simulink model "DR_ForceToTorque"  (R2022a)
settings: Solver=VariableStepAuto  StartTime=0.0  StopTime=10  RelTol=1e-3
undefined symbols (not defined in the file): X, Y, Z
libraries: sm_lib x9, nesl_utility x7
settings Model: Creator=bobjo  LastModifiedBy=bobjo

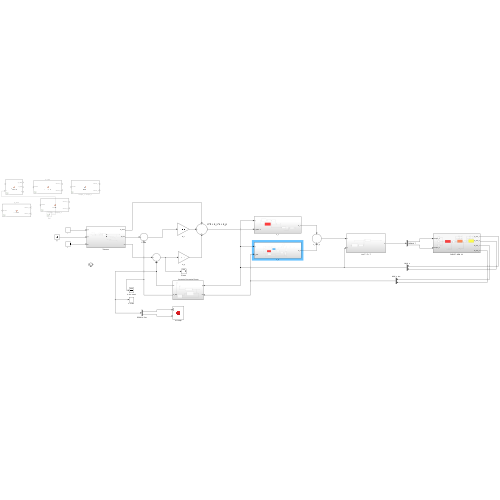
[thumbnail: Simulink's stored preview of the top-level diagram]
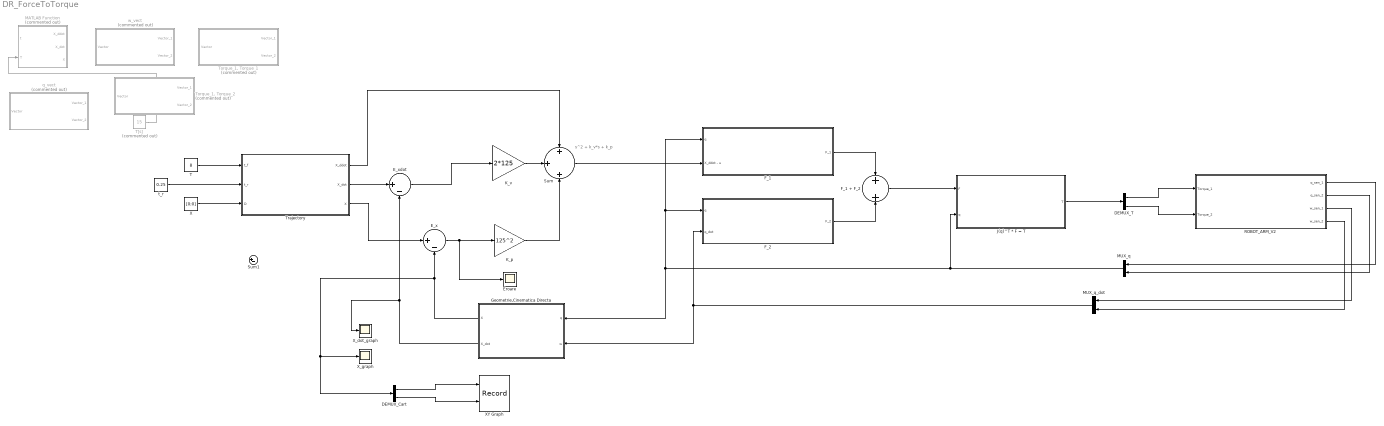
== system DR_ForceToTorque ==
  note: s^2 + k_v*s + k_p
  " MUX_q" : Mux  Inputs=2
  DEMUX_Cart : Demux  Outputs=2
  DEMUX_T : Demux  Outputs=2
  E_x : Sum  Inputs=|+-
  E_xdot : Sum  Inputs=|+-
  Eroare : Scope
  F_1 : Subsystem
  F_1 + F_2 : Sum  Inputs=+|+
  F_2 : Subsystem
  Geometrie,Cinematica Directa : Subsystem
  J(q)^T * F = T : Subsystem
  K_p : Gain  Gain=125^2
  K_v : Gain  Gain=2*125
  MATLAB Function : MATLAB Function  Commented=on  TreatAsAtomicUnit=on
  MUX_q_dot : Mux  Inputs=2
  ROBOT_ARM_V2 : Subsystem
  Sum : Sum  Inputs=+|+|+
  Sum1 : Sum  Inputs=|+-
  T : Constant  Value=8
  T[s] : Constant  Commented=on  Value=15
  "Torque_1, Torque_1" : MATLAB Function  Commented=on  TreatAsAtomicUnit=on
  "Torque_1, Torque_2" : MATLAB Function  Commented=on  TreatAsAtomicUnit=on
  Trajectory : Subsystem
  X : Constant  Value=[0;0]
  XY Graph : Record  FileSettingsInternal="{\"entries\":[{\"content\":{\"excelSettings\":{\"content\":{},\"type\":\"Streamout.ExcelSettings\"}},\"type\":\"Streamout.FileSettingStorage\",\"uuid\":\"b94b4cba-0fe7-4e66-af93-bfd95075920f\"}],\"packageUris\":[\"http://schema.mathworks.com/mf0/streamout_blocks/R2020a\"],\"version\":\"1.0\"}"  Layout=[1 1]  SignalsInternal="{\"entries\":[{\"content\":{\"signals\":[{\"content\":{\"blockPath\":[\"DR_ForceToTorque/XY Graph\"],\"channel\":[],\"dimensions\":[1,1],\"domain\":\"DR_ForceToTorque/XY Graph\",\"lineColor\":\"#a2142f\",\"plots\":[1],\"port\":1,\"sid\":[\"\"],\"signalID\":20,\"signalName\":\"DEMUX_Cart:1\"},\"type\":\"RecordBlkView.Signal\",\"uuid\":\"102e7f18-ab4c-4a7b-a2e7-68a635edeffb\"},{\"content\":{\"blockPath\":[\"DR_ForceToTorque/XY Graph\"],\"channel\":[],\"dimensions\":[1,1],\"domain\":\"DR_ForceToTorque/XY Graph\",\"lineColor\":\"#139fff\",\"plots\":[1],\"port\":2,\"sid\":[\"\"],\"signalID\":24,\"signalName\":\"DEMUX_Cart:2\"},\"type\":\"RecordBlkView.Signal\",\"uuid\":\"6c0b5dfe-2c0c-4a8d-93c7-f0d4dc18e998\"}]},\"type\":\"RecordBlkView.InputSignals\",\"uuid\":\"2a78a68b-d20b-47b5-ae5b-fe216d435864\"}],\"packageUris\":[\"http://schema.mathworks.com/mf0/streamout_blocks/R2020a\"],\"version\":\"1.0\"}"  VisualizationBindings="{\"xyplotplugin\":{\"info\":[{\"series\":[{\"bindingParametersList\":[{\"parameter\":\"X-Axis\",\"signalID\":20,\"signalName\":\"DEMUX_Cart:1\"},{\"parameter\":\"Y-Axis\",\"signalID\":24,\"signalName\":\"DEMUX_Cart:2\"}],\"seriesID\":43765}],\"subplotID\":1}]}}"  CompatibilityTag=XY
  X_dot_graph : Scope
  X_graph : Scope
  q_vect : MATLAB Function  Commented=on  TreatAsAtomicUnit=on
  t_r : Constant  Value=0.25
  w_vect : MATLAB Function  Commented=on  TreatAsAtomicUnit=on
  wires:
  F_1/1(F_1) -> F_1 + F_2/1
  F_2/1(F_2) -> F_1 + F_2/2
  F_1 + F_2/1 -> J(q)^T * F = T/1(F)
  Sum/1 -> F_1/2(X_ddot - u)
  E_x/1 -> Eroare/1, K_p/1
  E_xdot/1 -> K_v/1
  K_v/1 -> Sum/2
  K_p/1 -> Sum/3
  Geometrie,Cinematica Directa/2(X_dot) -> X_dot_graph/1, E_xdot/2
  Geometrie,Cinematica Directa/1(X) -> DEMUX_Cart/1, X_graph/1, E_x/2
  T[s]/1 -> MATLAB Function/2(T)
  T/1 -> Trajectory/1("t_f ")
  t_r/1 -> Trajectory/2("t_r ")
  Trajectory/1(X_ddot) -> Sum/1
  Trajectory/2(X_dot) -> E_xdot/1
  Trajectory/3(X) -> E_x/1
  J(q)^T * F = T/1(T) -> DEMUX_T/1
  DEMUX_T/1 -> ROBOT_ARM_V2/1(Torque_1)
  DEMUX_T/2 -> ROBOT_ARM_V2/2(Torque_2)
  ROBOT_ARM_V2/1(q_sen_1) -> " MUX_q"/1
  ROBOT_ARM_V2/2(q_sen_2) -> " MUX_q"/2
  ROBOT_ARM_V2/3(w_sen_1) -> MUX_q_dot/1
  ROBOT_ARM_V2/4(w_sen_2) -> MUX_q_dot/2
  " MUX_q"/1 -> Geometrie,Cinematica Directa/1(q), F_1/1(q), F_2/1(q), J(q)^T * F = T/2(q)
  MUX_q_dot/1 -> Geometrie,Cinematica Directa/2(w), F_2/2(q_dot)
  DEMUX_Cart/1 -> XY Graph/1
  DEMUX_Cart/2 -> XY Graph/2
  X/1 -> Trajectory/3(D)

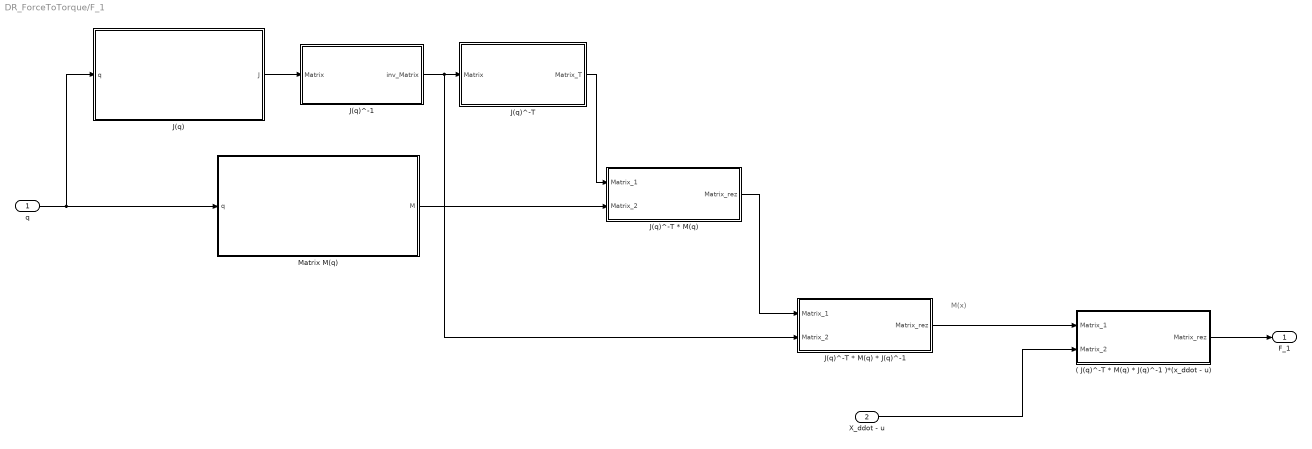
== system DR_ForceToTorque/F_1 ==
  note: M(x)
  q : Inport
  X_ddot - u : Inport  Port=2
  ( J(q)^-T * M(q) * J(q)^-1 )*(x_ddot - u) : MATLAB Function  TreatAsAtomicUnit=on
  J(q) : MATLAB Function  TreatAsAtomicUnit=on
  J(q)^-1 : MATLAB Function  TreatAsAtomicUnit=on
  J(q)^-T : MATLAB Function  TreatAsAtomicUnit=on
  J(q)^-T * M(q) : MATLAB Function  TreatAsAtomicUnit=on
  J(q)^-T * M(q) * J(q)^-1 : MATLAB Function  TreatAsAtomicUnit=on
  Matrix M(q) : MATLAB Function  TreatAsAtomicUnit=on
  F_1 : Outport
  wires:
  Matrix M(q)/1(M) -> J(q)^-T * M(q)/2(Matrix_2)
  J(q)/1(J) -> J(q)^-1/1(Matrix)
  J(q)^-1/1(inv_Matrix) -> J(q)^-T/1(Matrix), J(q)^-T * M(q) * J(q)^-1/2(Matrix_2)
  ( J(q)^-T * M(q) * J(q)^-1 )*(x_ddot - u)/1(Matrix_rez) -> F_1/1
  q/1 -> Matrix M(q)/1(q), J(q)/1(q)
  J(q)^-T * M(q)/1(Matrix_rez) -> J(q)^-T * M(q) * J(q)^-1/1(Matrix_1)
  J(q)^-T * M(q) * J(q)^-1/1(Matrix_rez) -> ( J(q)^-T * M(q) * J(q)^-1 )*(x_ddot - u)/1(Matrix_1)
  X_ddot - u/1 -> ( J(q)^-T * M(q) * J(q)^-1 )*(x_ddot - u)/2(Matrix_2)
  J(q)^-T/1(Matrix_T) -> J(q)^-T * M(q)/1(Matrix_1)

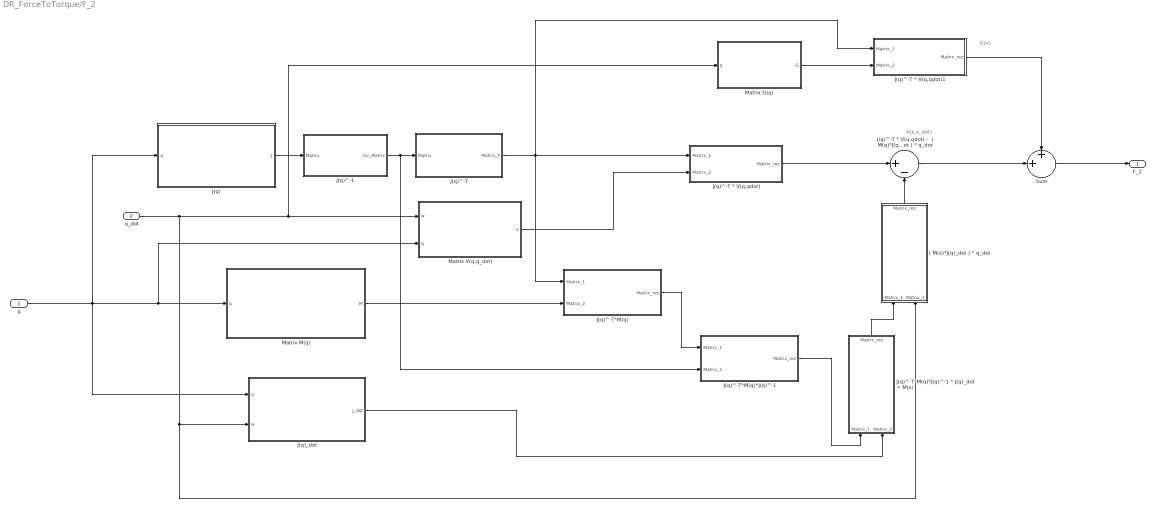
== system DR_ForceToTorque/F_2 ==
  note: G(x)
  note: V(x,x_dot)
  q : Inport
  q_dot : Inport  Port=2
  ( M(x)*J(q)_dot ) * q_dot : MATLAB Function  TreatAsAtomicUnit=on
  J(q) : MATLAB Function  TreatAsAtomicUnit=on
  J(q)^-1 : MATLAB Function  TreatAsAtomicUnit=on
  J(q)^-T : MATLAB Function  TreatAsAtomicUnit=on
  J(q)^-T * V(q,qdot) : MATLAB Function  TreatAsAtomicUnit=on
  J(q)^-T * V(q,qdot) -  ( M(q)*J(q)_dot ) * q_dot : Sum  Inputs=|+-
  J(q)^-T * V(q,qdot)1 : MATLAB Function  TreatAsAtomicUnit=on
  J(q)^-T*M(q) : MATLAB Function  TreatAsAtomicUnit=on
  J(q)^-T*M(q)*J(q)^-1 : MATLAB Function  TreatAsAtomicUnit=on
  J(q)^-T*M(q)*J(q)^-1 * J(q)_dot = M(x) : MATLAB Function  TreatAsAtomicUnit=on
  J(q)_dot : MATLAB Function  TreatAsAtomicUnit=on
  Matrix G(q) : MATLAB Function  TreatAsAtomicUnit=on
  Matrix M(q) : MATLAB Function  TreatAsAtomicUnit=on
  Matrix V(q,q_dot) : MATLAB Function  TreatAsAtomicUnit=on
  Sum : Sum  Inputs=++|
  F_2 : Outport
  wires:
  q/1 -> J(q)/1(q), J(q)_dot/1(q), Matrix V(q,q_dot)/2(q), Matrix M(q)/1(q)
  J(q)/1(J) -> J(q)^-1/1(Matrix)
  J(q)^-1/1(inv_Matrix) -> J(q)^-T/1(Matrix), J(q)^-T*M(q)*J(q)^-1/2(Matrix_2)
  J(q)^-T/1(Matrix_T) -> J(q)^-T * V(q,qdot)/1(Matrix_1), J(q)^-T * V(q,qdot)1/1(Matrix_1), J(q)^-T*M(q)/1(Matrix_1)
  Matrix V(q,q_dot)/1(V) -> J(q)^-T * V(q,qdot)/2(Matrix_2)
  q_dot/1 -> J(q)_dot/2(w), ( M(x)*J(q)_dot ) * q_dot/2(Matrix_2), Matrix G(q)/1(q), Matrix V(q,q_dot)/1(w)
  J(q)^-T * V(q,qdot)/1(Matrix_rez) -> J(q)^-T * V(q,qdot) -  ( M(q)*J(q)_dot ) * q_dot/1
  J(q)_dot/1(J_dot) -> J(q)^-T*M(q)*J(q)^-1 * J(q)_dot = M(x)/2(Matrix_2)
  J(q)^-T*M(q)*J(q)^-1 * J(q)_dot = M(x)/1(Matrix_rez) -> ( M(x)*J(q)_dot ) * q_dot/1(Matrix_1)
  ( M(x)*J(q)_dot ) * q_dot/1(Matrix_rez) -> J(q)^-T * V(q,qdot) -  ( M(q)*J(q)_dot ) * q_dot/2
  Matrix M(q)/1(M) -> J(q)^-T*M(q)/2(Matrix_2)
  J(q)^-T*M(q)/1(Matrix_rez) -> J(q)^-T*M(q)*J(q)^-1/1(Matrix_1)
  J(q)^-T*M(q)*J(q)^-1/1(Matrix_rez) -> J(q)^-T*M(q)*J(q)^-1 * J(q)_dot = M(x)/1(Matrix_1)
  Sum/1 -> F_2/1
  J(q)^-T * V(q,qdot) -  ( M(q)*J(q)_dot ) * q_dot/1 -> Sum/2
  Matrix G(q)/1(G) -> J(q)^-T * V(q,qdot)1/2(Matrix_2)
  J(q)^-T * V(q,qdot)1/1(Matrix_rez) -> Sum/1

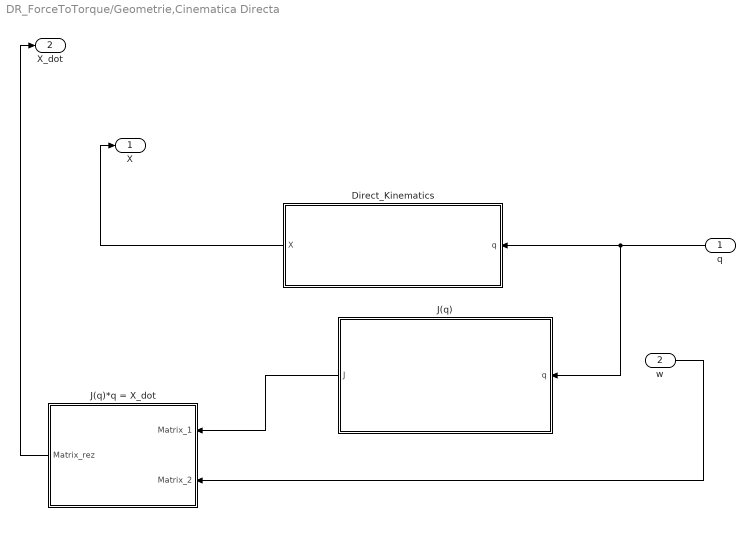
== system DR_ForceToTorque/Geometrie,Cinematica Directa ==
  q : Inport
  w : Inport  Port=2
  Direct_Kinematics : MATLAB Function  TreatAsAtomicUnit=on
  J(q) : MATLAB Function  TreatAsAtomicUnit=on
  J(q)*q = X_dot : MATLAB Function  TreatAsAtomicUnit=on
  X : Outport
  X_dot : Outport  Port=2
  wires:
  w/1 -> J(q)*q = X_dot/2(Matrix_2)
  Direct_Kinematics/1(X) -> X/1
  J(q)/1(J) -> J(q)*q = X_dot/1(Matrix_1)
  q/1 -> J(q)/1(q), Direct_Kinematics/1(q)
  J(q)*q = X_dot/1(Matrix_rez) -> X_dot/1

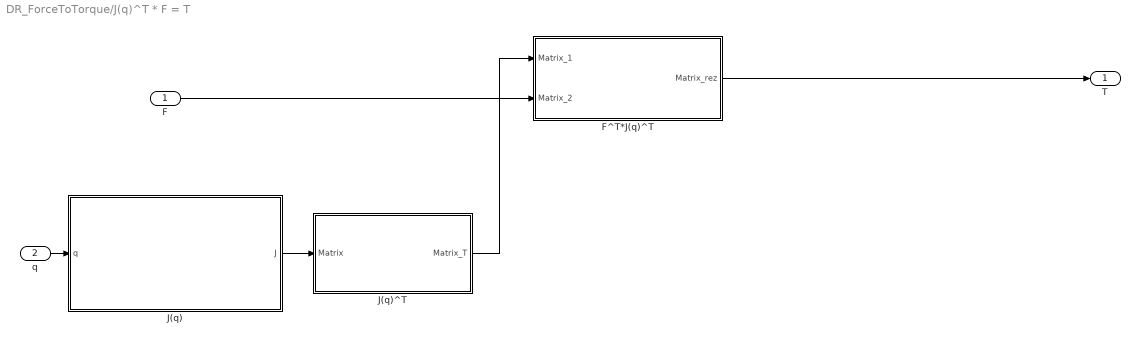
== system DR_ForceToTorque/J(q)^T * F = T ==
  F : Inport
  q : Inport  Port=2
  F^T*J(q)^T : MATLAB Function  TreatAsAtomicUnit=on
  J(q) : MATLAB Function  TreatAsAtomicUnit=on
  J(q)^T : MATLAB Function  TreatAsAtomicUnit=on
  T : Outport
  wires:
  J(q)/1(J) -> J(q)^T/1(Matrix)
  q/1 -> J(q)/1(q)
  J(q)^T/1(Matrix_T) -> F^T*J(q)^T/1(Matrix_1)
  F^T*J(q)^T/1(Matrix_rez) -> T/1
  F/1 -> F^T*J(q)^T/2(Matrix_2)

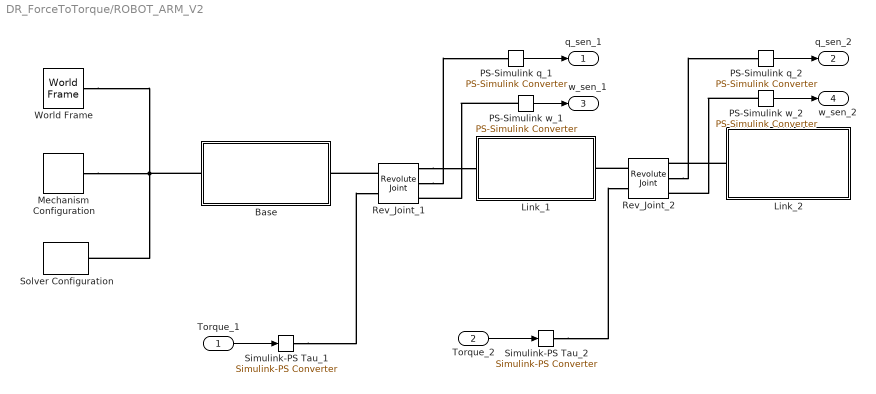
== system DR_ForceToTorque/ROBOT_ARM_V2 ==
  Torque_1 : Inport
  Torque_2 : Inport  Port=2
  Base : Subsystem
  Link_1 : Subsystem
  Link_2 : Subsystem
  Mechanism Configuration : sm_lib/Utilities/Mechanism Configuration  UniformGravity=Constant  GravityVector=[0 0 -9.80665]  GravityUnits=m/s^2  LinearizationDelta=0.001  JointModeTransitionNonlinearIterations=2
  PS-Simulink q_1 : nesl_utility/PS-Simulink Converter  PhysicalDomain=network_engine_domain  SubClassName=ps_output  LeftPortType=input  RightPortType=output  PseudoPeriodic=off  Frequencies=[]  VectorFormat=inherit  Unit=inherit  AffineConversion=off
      settings: SourceProductBaseCode=SS,PW,VE
  PS-Simulink q_2 : nesl_utility/PS-Simulink Converter  PhysicalDomain=network_engine_domain  SubClassName=ps_output  LeftPortType=input  RightPortType=output  PseudoPeriodic=off  Frequencies=[]  VectorFormat=inherit  Unit=inherit  AffineConversion=off
      settings: SourceProductBaseCode=SS,PW,VE
  PS-Simulink w_1 : nesl_utility/PS-Simulink Converter  PhysicalDomain=network_engine_domain  SubClassName=ps_output  LeftPortType=input  RightPortType=output  PseudoPeriodic=off  Frequencies=[]  VectorFormat=inherit  Unit=inherit  AffineConversion=off
      settings: SourceProductBaseCode=SS,PW,VE
  PS-Simulink w_2 : nesl_utility/PS-Simulink Converter  PhysicalDomain=network_engine_domain  SubClassName=ps_output  LeftPortType=input  RightPortType=output  PseudoPeriodic=off  Frequencies=[]  VectorFormat=inherit  Unit=inherit  AffineConversion=off
      settings: SourceProductBaseCode=SS,PW,VE
  Rev_Joint_1 : sm_lib/Joints/Revolute Joint  JointMode=Normal  SenseConstraintForce=off  SenseConstraintForceX=off  SenseConstraintForceY=off  SenseConstraintForceZ=off  SenseConstraintTorque=off  SenseConstraintTorqueX=off  SenseConstraintTorqueY=off  SenseConstraintTorqueZ=off  SenseTotalForce=off  SenseTotalForceX=off  SenseTotalForceY=off  SenseTotalForceZ=off  SenseTotalTorque=off  SenseTotalTorqueX=off  SenseTotalTorqueY=off  SenseTotalTorqueZ=off  CompositeWrenchDir=FollowerOnBase  CompositeWrenchFrame=BaseFrame  EquilibriumPosition=0  EquilibriumPositionUnits=deg  SpringStiffness=0  SpringStiffnessUnits=N*m/deg  DampingCoefficient=0  DampingCoefficientUnits=N*m/(deg/s)  TorqueActuationMode=InputTorque  MotionActuationMode=ComputedMotion  SensePosition=on  SenseVelocity=on  SenseAcceleration=off  SenseTorqueForce=off  SenseLowerLimitTorqueForce=off  SenseUpperLimitTorqueForce=off  LowerLimitSpecify=off  LowerLimitBound=-90  LowerLimitBoundUnits=deg  LowerLimitStiffness=1e4  LowerLimitStiffnessUnits=N*m/deg  LowerLimitDamping=10  LowerLimitDampingUnits=N*m/(deg/s)  LowerLimitTransitionRegionWidth=0.1  LowerLimitTransitionRegionWidthUnits=deg  UpperLimitSpecify=off  UpperLimitBound=90  UpperLimitBoundUnits=deg  UpperLimitStiffness=1e4  UpperLimitStiffnessUnits=N*m/deg  UpperLimitDamping=10  UpperLimitDampingUnits=N*m/(deg/s)  UpperLimitTransitionRegionWidth=0.1  UpperLimitTransitionRegionWidthUnits=deg  PositionTargetSpecify=on  PositionTargetPriority=High  PositionTargetValue=0  PositionTargetValueUnits=rad  VelocityTargetSpecify=off  VelocityTargetPriority=High  VelocityTargetValue=0  VelocityTargetValueUnits=deg/s
  Rev_Joint_2 : sm_lib/Joints/Revolute Joint  JointMode=Normal  SenseConstraintForce=off  SenseConstraintForceX=off  SenseConstraintForceY=off  SenseConstraintForceZ=off  SenseConstraintTorque=off  SenseConstraintTorqueX=off  SenseConstraintTorqueY=off  SenseConstraintTorqueZ=off  SenseTotalForce=off  SenseTotalForceX=off  SenseTotalForceY=off  SenseTotalForceZ=off  SenseTotalTorque=off  SenseTotalTorqueX=off  SenseTotalTorqueY=off  SenseTotalTorqueZ=off  CompositeWrenchDir=FollowerOnBase  CompositeWrenchFrame=BaseFrame  EquilibriumPosition=0  EquilibriumPositionUnits=deg  SpringStiffness=0  SpringStiffnessUnits=N*m/deg  DampingCoefficient=0  DampingCoefficientUnits=N*m/(deg/s)  TorqueActuationMode=InputTorque  MotionActuationMode=ComputedMotion  SensePosition=on  SenseVelocity=on  SenseAcceleration=off  SenseTorqueForce=off  SenseLowerLimitTorqueForce=off  SenseUpperLimitTorqueForce=off  LowerLimitSpecify=off  LowerLimitBound=-90  LowerLimitBoundUnits=deg  LowerLimitStiffness=1e4  LowerLimitStiffnessUnits=N*m/deg  LowerLimitDamping=10  LowerLimitDampingUnits=N*m/(deg/s)  LowerLimitTransitionRegionWidth=0.1  LowerLimitTransitionRegionWidthUnits=deg  UpperLimitSpecify=off  UpperLimitBound=90  UpperLimitBoundUnits=deg  UpperLimitStiffness=1e4  UpperLimitStiffnessUnits=N*m/deg  UpperLimitDamping=10  UpperLimitDampingUnits=N*m/(deg/s)  UpperLimitTransitionRegionWidth=0.1  UpperLimitTransitionRegionWidthUnits=deg  PositionTargetSpecify=on  PositionTargetPriority=High  PositionTargetValue=0  PositionTargetValueUnits=rad  VelocityTargetSpecify=off  VelocityTargetPriority=High  VelocityTargetValue=0  VelocityTargetValueUnits=deg/s
  Simulink-PS Tau_1 : nesl_utility/Simulink-PS Converter  PhysicalDomain=network_engine_domain  SubClassName=ps_input  LeftPortType=input  RightPortType=output  PseudoPeriodic=off  Frequencies=[]  NoiseDistribution=none  NoiseParameters=[]  Unit=N*m  AffineConversion=off  FilteringAndDerivatives=provide  SimscapeFilterOrder=2  InputFilterTimeConstant=0.001  UdotUserProvided=0
      settings: SourceProductBaseCode=SS,PW,VE
  Simulink-PS Tau_2 : nesl_utility/Simulink-PS Converter  PhysicalDomain=network_engine_domain  SubClassName=ps_input  LeftPortType=input  RightPortType=output  PseudoPeriodic=off  Frequencies=[]  NoiseDistribution=none  NoiseParameters=[]  Unit=N*m  AffineConversion=off  FilteringAndDerivatives=provide  SimscapeFilterOrder=2  InputFilterTimeConstant=0.001  UdotUserProvided=0
      settings: SourceProductBaseCode=SS,PW,VE
  Solver Configuration : nesl_utility/Solver Configuration  PhysicalDomain=network_engine_domain  SubClassName=solver  LeftPortType=input  RightPortType=generic  Tones=[]  Harmonics=[]  SimulateNoise=off  Profile=off  UseLocalSampling=off  EnableSwitchedLinearOptims=on  FrequencyDomain=off  UseCCode=off  RelTol=0.001  AbsTol=0.001  MinStep=1e-09  ToWorkspace=off  RevertToSquareIcSolve=off  NumHomotopyIterations=100  PhasorMode=off  PhasorModeNumHarmonics=1  IndexReductionMethod=DerivativeReplacement  DoDC=off  ResidualTolerance=1e-09  UseLocalSolver=off  LocalSolverChoice=NE_BACKWARD_EULER_ADVANCER  LocalSolverSampleTime=0.001  DoFixedCost=off  MaxNonlinIter=3  MaxModeIter=2  ComputeImpulses=off  ImpulseIterations=2  LinearAlgebra=auto  LinearAlgebraNumThread=0  EquationFormulation=NE_TIME_EF  DelaysMemoryBudget=1024  AutomaticFiltering=on  FilteringTimeConstant=0.001  PartitionStorageMethod=AS_NEEDED  PartitionMemoryBudget=1024  PartitionMethod=ROBUST
      settings: SourceProductBaseCode=SS,PW,VE
  World Frame : sm_lib/Frames and Transforms/World Frame
  q_sen_1 : Outport
  q_sen_2 : Outport  Port=2
  w_sen_1 : Outport  Port=3
  w_sen_2 : Outport  Port=4
  wires:
  Torque_1/1 -> Simulink-PS Tau_1/1
  Torque_2/1 -> Simulink-PS Tau_2/1
  PS-Simulink q_1/1 -> q_sen_1/1
  PS-Simulink q_2/1 -> q_sen_2/1
  PS-Simulink w_1/1 -> w_sen_1/1
  PS-Simulink w_2/1 -> w_sen_2/1
  connections:
  Rev_Joint_2/RConn2 -- PS-Simulink q_2/LConn1
  Simulink-PS Tau_1/RConn1 -- Rev_Joint_1/LConn2
  Simulink-PS Tau_2/RConn1 -- Rev_Joint_2/LConn2
  Mechanism Configuration/RConn1 -- Solver Configuration/RConn1 -- Base/LConn1 -- World Frame/RConn1
  Rev_Joint_1/LConn1 -- Base/RConn1
  Rev_Joint_1/RConn1 -- Link_1/LConn1
  Rev_Joint_2/LConn1 -- Link_1/RConn1
  Rev_Joint_1/RConn2 -- PS-Simulink q_1/LConn1
  Link_2/RConn1 -- Rev_Joint_2/RConn1
  PS-Simulink w_2/LConn1 -- Rev_Joint_2/RConn3
  PS-Simulink w_1/LConn1 -- Rev_Joint_1/RConn3

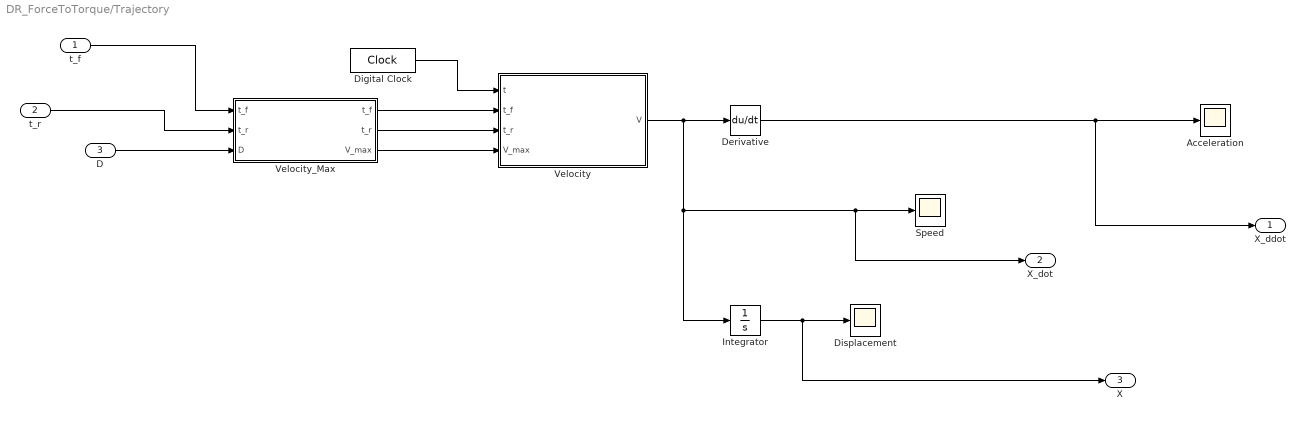
== system DR_ForceToTorque/Trajectory ==
  "t_f " : Inport
  "t_r " : Inport  Port=2
  D : Inport  Port=3
  Acceleration : Scope
  Derivative : Derivative
  Digital Clock : DigitalClock  SampleTime=0.001
  Displacement : Scope
  Integrator : Integrator  InitialCondition=[1;0]
  Speed : Scope
  Velocity : MATLAB Function  TreatAsAtomicUnit=on
  Velocity_Max : MATLAB Function  TreatAsAtomicUnit=on
  X_ddot : Outport
  X_dot : Outport  Port=2
  X : Outport  Port=3
  wires:
  Velocity/1(V) -> X_dot/1, Speed/1, Integrator/1, Derivative/1
  Digital Clock/1 -> Velocity/1(t)
  Integrator/1 -> Displacement/1, X/1
  Derivative/1 -> Acceleration/1, X_ddot/1
  "t_f "/1 -> Velocity_Max/1("t_f ")
  Velocity_Max/1(t_f) -> Velocity/2(t_f)
  Velocity_Max/3(V_max) -> Velocity/4(V_max)
  "t_r "/1 -> Velocity_Max/2("t_r ")
  Velocity_Max/2(t_r) -> Velocity/3(t_r)
  D/1 -> Velocity_Max/3(D)

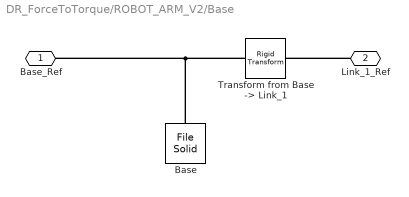
== system DR_ForceToTorque/ROBOT_ARM_V2/Base ==
  Base : sm_lib/Body Elements/File Solid  ExtGeomFileName=C:\Users\bobjo\OneDrive\Desktop\Facultate ROBO\Anul III\DR\Base_V2.CATPart  UnitType=FromFile  ExtGeomFileUnits=m  StepReaderType=HEX  ExportConvexHullGeometry=off  InertiaType=CalculateFromGeometry  Mass=1  MassUnits=kg  CenterOfMass=[0 0 0]  CenterOfMassUnits=m  MomentsOfInertia=[1 1 1]  MomentsOfInertiaUnits=kg*m^2  ProductsOfInertia=[0 0 0]  ProductsOfInertiaUnits=kg*m^2  BasedOnType=DensityFromFile  Density=1000  DensityUnits=kg/m^3  DoExposeReferenceFrame=on  SerializedFrames=<Frames/>  GraphicType=FromGeometry  MarkerShape=Sphere  MarkerSize=10  GraphicVisPropType=SimpleVisualProperties  GraphicDiffuseColor=[1.0 0.0 0.2]  GraphicSpecularColor=[0.5 0.5 0.5 1.0]  GraphicAmbientColor=[0.15 0.15 0.15 1.0]  GraphicEmissiveColor=[0.0 0.0 0.0 1.0]  GraphicShininess=75  GraphicOpacity=1.0
  "Transform from Base -> Link_1" : sm_lib/Frames and Transforms/Rigid Transform  TranslationMethod=Cartesian  TranslationStandardOffset=0  TranslationLengthUnit=mm  TranslationStandardAxis=+Z  TranslationCartesianOffset=[0 0 40]  TranslationROffset=0  TranslationROffsetUnits=m  TranslationZOffset=0  TranslationZOffsetUnits=m  TranslationThetaOffset=0  TranslationThetaOffsetUnits=deg  RotationMethod=None  RotationAngleUnits=deg  RotationStandardAxis=+Z  RotationAngle=0.0  RotationArbitraryAxis=[0 0 1]  FollAlignAxisA=+X  BaseAlignAxisA=+Y  FollAlignAxisB=+Y  BaseAlignAxisB=+Z  RotationSequenceAxes=FollowerAxes  RotationSequence=XYX  RotationSequenceAngles=[0 0 0]  RotationSequenceAnglesUnits=deg  RotationMatrix=[1 0 0; 0 1 0; 0 0 1]
  Base_Ref : PMIOPort  Side=Left
  Link_1_Ref : PMIOPort  Port=2  Side=Right
  connections:
  Base/RConn1 -- Base_Ref/RConn1 -- "Transform from Base -> Link_1"/LConn1
  Link_1_Ref/RConn1 -- "Transform from Base -> Link_1"/RConn1

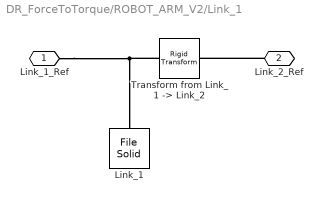
== system DR_ForceToTorque/ROBOT_ARM_V2/Link_1 ==
  Link_1 : sm_lib/Body Elements/File Solid  ExtGeomFileName=C:\Users\bobjo\OneDrive\Desktop\Facultate ROBO\Anul III\DR\Link_1_V2.CATPart  UnitType=FromFile  ExtGeomFileUnits=m  StepReaderType=HEX  ExportConvexHullGeometry=off  InertiaType=CalculateFromGeometry  Mass=0.25  MassUnits=kg  CenterOfMass=[0 0 0]  CenterOfMassUnits=m  MomentsOfInertia=[1 1 1]  MomentsOfInertiaUnits=kg*m^2  ProductsOfInertia=[0 0 0]  ProductsOfInertiaUnits=kg*m^2  BasedOnType=DensityFromFile  Density=1000  DensityUnits=kg/m^3  DoExposeReferenceFrame=on  SerializedFrames=<Frames/>  GraphicType=FromGeometry  MarkerShape=Sphere  MarkerSize=10  GraphicVisPropType=SimpleVisualProperties  GraphicDiffuseColor=[1.0 0.4 0.0]  GraphicSpecularColor=[0.5 0.5 0.5 1.0]  GraphicAmbientColor=[0.15 0.15 0.15 1.0]  GraphicEmissiveColor=[0.0 0.0 0.0 1.0]  GraphicShininess=75  GraphicOpacity=1.0
  "Transform from Link_1 -> Link_2" : sm_lib/Frames and Transforms/Rigid Transform  TranslationMethod=Cartesian  TranslationStandardOffset=0  TranslationLengthUnit=mm  TranslationStandardAxis=+Z  TranslationCartesianOffset=[500 0 50]  TranslationROffset=0  TranslationROffsetUnits=m  TranslationZOffset=0  TranslationZOffsetUnits=m  TranslationThetaOffset=0  TranslationThetaOffsetUnits=deg  RotationMethod=None  RotationAngleUnits=deg  RotationStandardAxis=+Z  RotationAngle=0.0  RotationArbitraryAxis=[0 0 1]  FollAlignAxisA=+X  BaseAlignAxisA=+Y  FollAlignAxisB=+Y  BaseAlignAxisB=+Z  RotationSequenceAxes=FollowerAxes  RotationSequence=XYX  RotationSequenceAngles=[0 0 0]  RotationSequenceAnglesUnits=deg  RotationMatrix=[1 0 0; 0 1 0; 0 0 1]
  Link_1_Ref : PMIOPort  Side=Left
  Link_2_Ref : PMIOPort  Port=2  Side=Right
  connections:
  Link_2_Ref/RConn1 -- "Transform from Link_1 -> Link_2"/RConn1
  "Transform from Link_1 -> Link_2"/LConn1 -- Link_1_Ref/RConn1 -- Link_1/RConn1

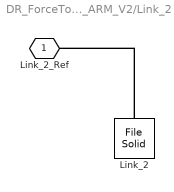
== system DR_ForceToTorque/ROBOT_ARM_V2/Link_2 ==
  Link_2 : sm_lib/Body Elements/File Solid  ExtGeomFileName=C:\Users\bobjo\OneDrive\Desktop\Facultate ROBO\Anul III\DR\Link_2_V2.CATPart  UnitType=FromFile  ExtGeomFileUnits=m  StepReaderType=HEX  ExportConvexHullGeometry=off  InertiaType=CalculateFromGeometry  Mass=0.25  MassUnits=kg  CenterOfMass=[0 0 0]  CenterOfMassUnits=m  MomentsOfInertia=[1 1 1]  MomentsOfInertiaUnits=kg*m^2  ProductsOfInertia=[0 0 0]  ProductsOfInertiaUnits=kg*m^2  BasedOnType=DensityFromFile  Density=1000  DensityUnits=kg/m^3  DoExposeReferenceFrame=on  SerializedFrames=<Frames/>  GraphicType=FromGeometry  MarkerShape=Sphere  MarkerSize=10  GraphicVisPropType=SimpleVisualProperties  GraphicDiffuseColor=[1.0 1.0 0.0]  GraphicSpecularColor=[0.5 0.5 0.5 1.0]  GraphicAmbientColor=[0.15 0.15 0.15 1.0]  GraphicEmissiveColor=[0.0 0.0 0.0 1.0]  GraphicShininess=75  GraphicOpacity=1.0
  Link_2_Ref : PMIOPort  Side=Right
  connections:
  Link_2/RConn1 -- Link_2_Ref/RConn1

== matlab function DR_ForceToTorque/F_2/J(q)^-T * V(q,qdot) ==
  data: Matrix_1 input; Matrix_rez output; Matrix_2 input
function Matrix_rez = Matrix_Multiply(Matrix_1,Matrix_2)

Matrix_rez = Matrix_1*Matrix_2;

== matlab function DR_ForceToTorque/F_2/J(q)_dot ==
  data: q input; J_dot output; w input
function J_dot = Jacobian_dot(q,w)

l_1 = 0.5;
l_2 = 0.5;
alfa = 0.01;

J_dot = [ -l_1*cos(q(1,:))*w(1,:) - l_2*cos(q(1,:) + q(2,:) + alfa)*(w(1,:)+w(2,:)), -l_2*cos(q(1,:) + q(2,:) + alfa)*(w(1,:)+w(2,:));
          -l_1*sin(q(1,:))*w(1,:) - l_2*sin(q(1,:) + q(2,:) + alfa)*(w(1,:)+w(2,:)), -l_2*sin(q(1,:) + q(2,:) + alfa)*(w(1,:)+w(2,:))];

== matlab function DR_ForceToTorque/F_2/J(q)^-T*M(q)*J(q)^-1 * J(q)_dot = M(x) ==
  data: Matrix_1 input; Matrix_rez output; Matrix_2 input
function Matrix_rez = Matrix_Multiply(Matrix_1,Matrix_2)

Matrix_rez = Matrix_1*Matrix_2;

== matlab function DR_ForceToTorque/F_1/J(q) ==
  data: q input; J output
function J = Jacobian(q)

l_1 = 0.5;
l_2 = 0.5;
alfa = 0.01;

J = [ -l_1*sin(q(1,:)) - l_2*sin(q(1,:) + q(2,:) + alfa ), -l_2*sin(q(1,:) + q(2,:) + alfa);
       l_1*cos(q(1,:)) + l_2*cos(q(1,:) + q(2,:) + alfa),   l_2*cos(q(1,:) + q(2,:) + alfa)];

== matlab function DR_ForceToTorque/F_2/( M(x)*J(q)_dot ) * q_dot ==
  data: Matrix_1 input; Matrix_rez output; Matrix_2 input
function Matrix_rez = Matrix_Multiply(Matrix_1,Matrix_2)

Matrix_rez = Matrix_1*Matrix_2;

== matlab function DR_ForceToTorque/MATLAB Function ==
  data: X_ddot output; X_dot output; t input; X output; T input
function [X_ddot,X_dot,X] = Trajectory(t,T)

x = 0;
y = 1;

X = ([x;y]-[1;0])*(-2*(t/T)^3+3*(t/T)^2)+[1;0];
X_dot = ([x;y]-[1;0])*(-6*t^2/T^3+6*t/T^2)+[1;0];
X_ddot = ([x;y]-[1;0])*(-12*t/T^3+6/T^2)+[1;0];

== matlab function DR_ForceToTorque/J(q)^T * F = T/J(q)^T ==
  data: Matrix input; Matrix_T output
function Matrix_T = transpose(Matrix)

Matrix_T = transpose(Matrix);

== matlab function DR_ForceToTorque/J(q)^T * F = T/F^T*J(q)^T ==
  data: Matrix_1 input; Matrix_rez output; Matrix_2 input
function Matrix_rez = Matrix_Multiply(Matrix_1,Matrix_2)

Matrix_rez = Matrix_1*Matrix_2;

== matlab function DR_ForceToTorque/Torque_1, Torque_2 ==
  data: Vector input; Vector_1 output; Vector_2 output
function [Vector_1,Vector_2] = divider(Vector)

Vector_1 = Vector(1,:);
Vector_2 = Vector(2,:);

== matlab function DR_ForceToTorque/q_vect ==
  data: Vector_1 input; Vector output; Vector_2 input
function Vector = combiner(Vector_1,Vector_2)

Vector = [Vector_1; Vector_2];

== matlab function DR_ForceToTorque/w_vect ==
  data: Vector_1 input; Vector output; Vector_2 input
function Vector = combiner(Vector_1,Vector_2)

Vector = [Vector_1; Vector_2];

== matlab function DR_ForceToTorque/Geometrie,Cinematica Directa/Direct_Kinematics ==
  data: q input; X output
function X = Dir_K(q)
l_1 = 0.5;
l_2 = 0.5;
X = [l_1*cos(q(1,:))+l_2*cos(q(1,:) + q(2,:)); l_1*sin(q(1,:))+l_2*sin(q(1,:) + q(2,:))];

== matlab function DR_ForceToTorque/F_2/J(q) ==
  data: q input; J output
function J = Jacobian(q)

l_1 = 0.5;
l_2 = 0.5;
alfa = 0.01;

J = [ -l_1*sin(q(1,:)) - l_2*sin(q(1,:) + q(2,:) + alfa ), -l_2*sin(q(1,:) + q(2,:) + alfa);
       l_1*cos(q(1,:)) + l_2*cos(q(1,:) + q(2,:) + alfa),   l_2*cos(q(1,:) + q(2,:) + alfa)];

== matlab function DR_ForceToTorque/F_1/J(q)^-1 ==
  data: Matrix input; inv_Matrix output
function inv_Matrix = Inverse (Matrix)

inv_Matrix = inv(Matrix);

== matlab function DR_ForceToTorque/Geometrie,Cinematica Directa/J(q)*q = X_dot ==
  data: Matrix_1 input; Matrix_rez output; Matrix_2 input
function Matrix_rez = Matrix_Multiply(Matrix_1,Matrix_2)

Matrix_rez = Matrix_1*Matrix_2;

== matlab function DR_ForceToTorque/Trajectory/Velocity_Max ==
  data: t_f output; t_r output; V_max output; t_f input; t_r input; D input
function [t_f,t_r,V_max] = Velocity_Max(t_f,t_r,D)

V_max = (D-[1;0])/(t_f-t_r);

== matlab function DR_ForceToTorque/Trajectory/Velocity ==
  data: t input; t_f input; t_r input; V output; V_max input
function V= Velocity(t,t_f,t_r,V_max)

V = [0;0];
if t <= t_r
    V = V_max*t/t_r;
end

if (t > t_r) && (t < t_f - t_r)
    V = V_max;
end

if (t >= t_f - t_r) && (t <= t_f)
    V = V_max*(t_f - t)/t_r;
end

== matlab function DR_ForceToTorque/Geometrie,Cinematica Directa/J(q) ==
  data: q input; J output
function J = Jacobian(q)

l_1 = 0.5;
l_2 = 0.5;
alfa = 0.01;

J = [ -l_1*sin(q(1,:)) - l_2*sin(q(1,:) + q(2,:) + alfa ), -l_2*sin(q(1,:) + q(2,:) + alfa);
       l_1*cos(q(1,:)) + l_2*cos(q(1,:) + q(2,:) + alfa),   l_2*cos(q(1,:) + q(2,:) + alfa)];

== matlab function DR_ForceToTorque/Torque_1, Torque_1 ==
  data: Vector input; Vector_1 output; Vector_2 output
function [Vector_1,Vector_2] = divider(Vector)

Vector_1 = Vector(1,:);
Vector_2 = Vector(2,:);

== matlab function DR_ForceToTorque/F_2/J(q)^-T*M(q) ==
  data: Matrix_1 input; Matrix_rez output; Matrix_2 input
function Matrix_rez = Matrix_Multiply(Matrix_1,Matrix_2)

Matrix_rez = Matrix_1*Matrix_2;

== matlab function DR_ForceToTorque/F_2/Matrix G(q) ==
  data: q input; G output
function G = G_Torque(q)

l_1 = 0.5;
l_2 = 0.5;

m_1 = 0.469;
m_2 = 0.51;

g = [0;0;9.8165];


J_v1 = [-l_1*sin(q(1,:)), 0;
         l_2*cos(q(1,:)), 0;
         0, 0];

J_v2 = [-l_1*sin(q(1,:))-l_2*sin(q(1,:)+q(2,:)), -l_2*sin(q(1,:)+q(2,:));
         l_1*cos(q(1,:))+l_2*cos(q(1,:)+q(2,:)),  l_2*cos(q(1,:)+q(2,:));
         0, 0];


G = [transpose(J_v1),transpose(J_v2)]*[m_1*g;m_2*g];

== matlab function DR_ForceToTorque/F_2/J(q)^-T * V(q,qdot)1 ==
  data: Matrix_1 input; Matrix_rez output; Matrix_2 input
function Matrix_rez = Matrix_Multiply(Matrix_1,Matrix_2)

Matrix_rez = Matrix_1*Matrix_2;

== matlab function DR_ForceToTorque/F_1/J(q)^-T * M(q) ==
  data: Matrix_1 input; Matrix_rez output; Matrix_2 input
function Matrix_rez = Matrix_Multiply(Matrix_1,Matrix_2)

Matrix_rez = Matrix_1*Matrix_2;

== matlab function DR_ForceToTorque/F_2/J(q)^-T*M(q)*J(q)^-1 ==
  data: Matrix_1 input; Matrix_rez output; Matrix_2 input
function Matrix_rez = Matrix_Multiply(Matrix_1,Matrix_2)

Matrix_rez = Matrix_1*Matrix_2;

== matlab function DR_ForceToTorque/F_1/J(q)^-T * M(q) * J(q)^-1 ==
  data: Matrix_1 input; Matrix_rez output; Matrix_2 input
function Matrix_rez = Matrix_Multiply(Matrix_1,Matrix_2)

Matrix_rez = Matrix_1*Matrix_2;

== matlab function DR_ForceToTorque/F_1/( J(q)^-T * M(q) * J(q)^-1 )*(x_ddot - u) ==
  data: Matrix_1 input; Matrix_rez output; Matrix_2 input
function Matrix_rez = Matrix_Multiply(Matrix_1,Matrix_2)

Matrix_rez = Matrix_1*Matrix_2;

== matlab function DR_ForceToTorque/F_2/Matrix M(q) ==
  data: M output; q input
function M = Inertial_Torque(q)

m_1 = 0.469;
m_2 = 0.51;

l_1 = 0.5;
l_2 = 0.5;
c_1 = l_1/2;
c_2 = l_2/2;

I_zz_1 = 0.011;
I_zz_2 = 0.013;

M = [ m_1*c_1^2 + m_2*(l_1^2 + c_2^2) + 2*m_2*l_1*c_2*cos(q(2,:)) + I_zz_1 + I_zz_2 , m_2*c_2^2 + m_2*l_1*c_2*cos(q(2,:)) + I_zz_2 ;
              m_2*c_2^2 + m_2*l_1*c_2*cos(q(2,:)) + I_zz_2                          ,           m_2*c_2^2 + I_zz_2              ];

== matlab function DR_ForceToTorque/J(q)^T * F = T/J(q) ==
  data: q input; J output
function J = Jacobian(q)

l_1 = 0.5;
l_2 = 0.5;
alfa = 0.01;

J = [ -l_1*sin(q(1,:)) - l_2*sin(q(1,:) + q(2,:) + alfa ), -l_2*sin(q(1,:) + q(2,:) + alfa);
       l_1*cos(q(1,:)) + l_2*cos(q(1,:) + q(2,:) + alfa),   l_2*cos(q(1,:) + q(2,:) + alfa)];

== matlab function DR_ForceToTorque/F_1/J(q)^-T ==
  data: Matrix input; Matrix_T output
function Matrix_T = transpose(Matrix)

Matrix_T = transpose(Matrix);

== matlab function DR_ForceToTorque/F_1/Matrix M(q) ==
  data: M output; q input
function M = Inertial_Torque(q)

m_1 = 0.469;
m_2 = 0.51;

l_1 = 0.5;
l_2 = 0.5;
c_1 = l_1/2;
c_2 = l_2/2;

I_zz_1 = 0.011;
I_zz_2 = 0.013;

M = [ m_1*c_1^2 + m_2*(l_1^2 + c_2^2) + 2*m_2*l_1*c_2*cos(q(2,:)) + I_zz_1 + I_zz_2 , m_2*c_2^2 + m_2*l_1*c_2*cos(q(2,:)) + I_zz_2 ;
              m_2*c_2^2 + m_2*l_1*c_2*cos(q(2,:)) + I_zz_2                          ,           m_2*c_2^2 + I_zz_2              ];

== matlab function DR_ForceToTorque/F_2/Matrix V(q,q_dot) ==
  data: w input; V output; q input
function  V= V_Torque(w,q)

m_2 = 0.51;

l_1 = 0.5;
l_2 = 0.5;
c_2 = l_2/2;

V = [-m_2*l_1*c_2*sin(q(2,:))*w(2,:)^2 - 2*m_2*l_1*c_2*sin(q(2,:))*w(1,:)*w(2,:);
                 m_2*l_1*c_2*sin(q(2,:))*w(1,:)^2                      ];

== matlab function DR_ForceToTorque/F_2/J(q)^-1 ==
  data: Matrix input; inv_Matrix output
function inv_Matrix = Inverse(Matrix)

inv_Matrix = inv(Matrix);

== matlab function DR_ForceToTorque/F_2/J(q)^-T ==
  data: Matrix input; Matrix_T output
function Matrix_T = transpose(Matrix)

Matrix_T = transpose(Matrix);
